simulink model "DC_motor"  (R2017a)
settings: Solver=VariableStepAuto  StartTime=0.0  StopTime=120  RelTol=1e-3
settings Model: Creator=Michy  LastModifiedBy=Michy

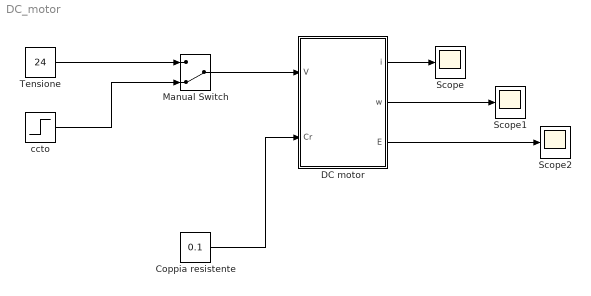
== system DC_motor ==
  Coppia resistente : Constant  Value=0.1
  DC motor : Subsystem  mask{L=0.0028, R=5.5, k=1, phi=0.5, J=0.5}
  Manual Switch : ManualSwitch  CurrentSetting=0
  Scope : Scope
  Scope1 : Scope
  Scope2 : Scope
  Tensione : Constant  Value=24
  ccto : Step  Time=60  Before=24  After=0  SampleTime=0
  wires:
  Coppia resistente/1 -> DC motor/2(Cr)
  DC motor/2(w) -> Scope1/1
  DC motor/1(i) -> Scope/1
  DC motor/3(E) -> Scope2/1
  Tensione/1 -> Manual Switch/1
  ccto/1 -> Manual Switch/2
  Manual Switch/1 -> DC motor/1(V)

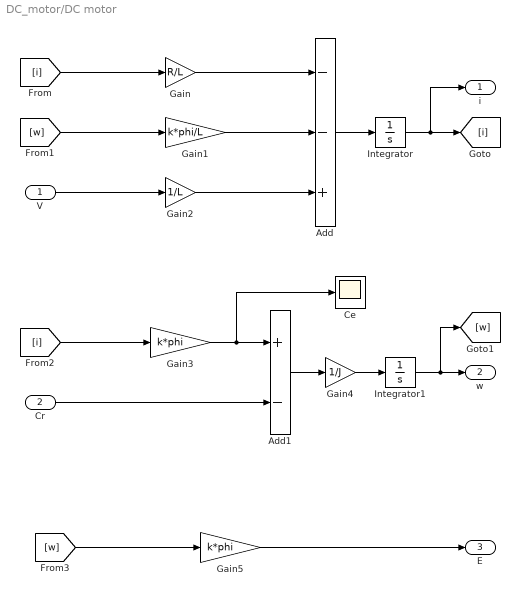
== system DC_motor/DC motor ==
  V : Inport
  Cr : Inport  Port=2
  Add : Sum  Inputs=--+
  Add1 : Sum  Inputs=+-
  Ce : Scope
  Gain : Gain  Gain=R/L
  Gain1 : Gain  Gain=k*phi/L
  Gain2 : Gain  Gain=1/L
  Gain3 : Gain  Gain=k*phi
  Gain4 : Gain  Gain=1/J
  Gain5 : Gain  Gain=k*phi
  Integrator : Integrator
  Integrator1 : Integrator
  i : Outport
  w : Outport  Port=2
  E : Outport  Port=3
  wires:
  [i] -> Gain/1
  [w] -> Gain1/1
  V/1 -> Gain2/1
  Gain/1 -> Add/1
  Gain1/1 -> Add/2
  Gain2/1 -> Add/3
  Add/1 -> Integrator/1
  Integrator/1 -> i/1, [i]
  [i] -> Gain3/1
  Gain3/1 -> Ce/1, Add1/1
  Cr/1 -> Add1/2
  Add1/1 -> Gain4/1
  Gain4/1 -> Integrator1/1
  Integrator1/1 -> [w], w/1
  [w] -> Gain5/1
  Gain5/1 -> E/1
